simulink model "EXP_Controller_YAW"  (R2015b)
settings: Solver=FixedStepAuto  StartTime=0.0  StopTime=inf  FixedStep=0.1  RelTol=1e-3
values from neighbouring files (symbols this model uses):
  breakpoints1 = data(end:-1:1,1)'    [Experimental_Impl.m]    (also in Experimental_Impl_wPlot.m; FEB02_LAKE_TEST.m; FEB14_LAKE_TEST.m; FEB28_LAKE_TEST.m)
  drag_coeff = 16.91    [Experimental_Impl.m]    (also in Experimental_Impl_wPlot.m; FEB02_LAKE_TEST.m = 8.5; FEB02_Post_Processing.m; FEB14_LAKE_TEST.m)
  Kdy = .1    (= 0.1)    [Experimental_Impl.m]    (also in Experimental_Impl_wPlot.m = Gain(3,i); FEB02_LAKE_TEST.m = 20; FEB02_Post_Processing.m = Gain_Y(3,k); FEB14_LAKE_TEST.m = 20)
  Kiy = .01    (= 0.01)    [Experimental_Impl.m]    (also in Experimental_Impl_wPlot.m = Gain(2,i); FEB02_LAKE_TEST.m; FEB02_Post_Processing.m = Gain_Y(2,k); FEB14_LAKE_TEST.m)
  Kpy = 1    [Experimental_Impl.m]    (also in Experimental_Impl_wPlot.m = Gain(1,i); FEB02_LAKE_TEST.m = 100; FEB02_Post_Processing.m = Gain_Y(1,k); FEB14_LAKE_TEST.m = 100)
  switch_case = 0    [Experimental_Impl.m]    (also in Experimental_Impl_wPlot.m; FEB02_LAKE_TEST.m = 1; FEB02_Post_Processing.m; FEB14_LAKE_TEST.m)
  table_data = data(end:-1:1,2)'    [Experimental_Impl.m]    (also in Experimental_Impl_wPlot.m; FEB02_LAKE_TEST.m; FEB14_LAKE_TEST.m; FEB28_LAKE_TEST.m)
  vf = 0.0    (= 0)    [Experimental_Impl.m]    (also in Experimental_Impl_wPlot.m; FEB02_LAKE_TEST.m = 1.5; FEB02_Post_Processing.m = 1.25; FEB14_LAKE_TEST.m = 1.5)
  vo = 0.0    (= 0)    [Experimental_Impl.m]    (also in Experimental_Impl_wPlot.m; FEB02_LAKE_TEST.m = 1.25; FEB02_Post_Processing.m = 1.25; FEB14_LAKE_TEST.m = 1.25)
  yf = pi/4    (= 0.785398163397)    [Experimental_Impl.m]    (also in Experimental_Impl_wPlot.m = 0; FEB02_LAKE_TEST.m = 0; FEB02_Post_Processing.m = pi()/4; FEB14_LAKE_TEST.m = 0)
  yo = 0    [Experimental_Impl.m]    (also in Experimental_Impl_wPlot.m; FEB02_LAKE_TEST.m; FEB02_Post_Processing.m; FEB14_LAKE_TEST.m)
undefined symbols (not defined in the file or in its folder): Left, Right
libraries: robotlib x3, simulink_extras x3, realtime_pacer_lib x1
settings Model: Creator=bsb  LastModifiedBy=aschnieders22
settings ConfigComp: CovModelRefEnable=Off

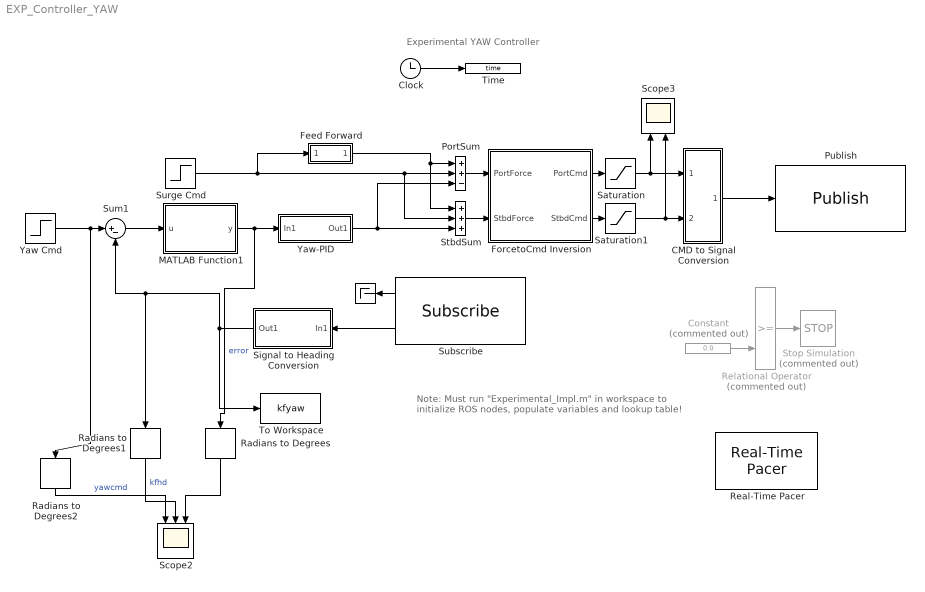
== system EXP_Controller_YAW ==
  note: Note: Must run "Experimental_Impl.m" in workspace to initialize ROS nodes, populate variables and lookup table!
  note: Experimental YAW Controller
  " " : Terminator
  CMD to Signal Conversion : Subsystem
  Clock : Clock
  Constant : Constant  Commented=on  Value=0.0
  Feed Forward : Subsystem
  ForcetoCmd Inversion : Subsystem
  MATLAB Function1 : MATLAB Function  TreatAsAtomicUnit=on
  PortSum : Sum  Inputs=++-
  Publish : robotlib/Publish  SourceLibraryInfo=This block requires Robotics System Toolbox  topicSource=Select from ROS network  topic=/cmd_drive  messageType=kingfisher_msgs/Drive  messageQueueLength=1
  Radians to Degrees : simulink_extras/Transformations/Radians to Degrees
  Radians to Degrees1 : simulink_extras/Transformations/Radians to Degrees
  Radians to Degrees2 : simulink_extras/Transformations/Radians to Degrees
  Real-Time Pacer : realtime_pacer_lib/Real-Time Pacer  simTimePerRealTime=1
  Relational Operator : RelationalOperator  Commented=on  OutDataTypeStr=boolean
  Saturation : Saturate  UpperLimit=1  LowerLimit=-1
  Saturation1 : Saturate  UpperLimit=1  LowerLimit=-1
  Scope2 : Scope  NumInputPorts=3
  Scope3 : Scope  NumInputPorts=2
  Signal to Heading Conversion : Subsystem
  StbdSum : Sum  Inputs=+++
  Stop Simulation : Stop  Commented=on
  Subscribe : robotlib/Subscribe  SourceLibraryInfo=This block requires Robotics System Toolbox  topicSource=Select from ROS network  topic=/imu/data  messageType=sensor_msgs/Imu  sampleTime=-1  messageQueueLength=1
  Sum1 : Sum  Inputs=|+-
  Surge Cmd : Step  Before=vo  After=vf  SampleTime=0
  Time : ToWorkspace  VariableName=time  SampleTime=-1
  To Workspace : ToWorkspace  VariableName=kfyaw  SampleTime=-1
  Yaw Cmd : Step  Time=0  Before=yo  After=yf  SampleTime=0
  Yaw-PID : Subsystem
  wires:
  Clock/1 -> Time/1
  CMD to Signal Conversion/1(Out1) -> Publish/1
  Feed Forward/1(Out1) -> PortSum/1, StbdSum/1
  Saturation1/1 -> Scope3/2, CMD to Signal Conversion/2(In2)
  Saturation/1 -> Scope3/1, CMD to Signal Conversion/1(In1)
  ForcetoCmd Inversion/2(StbdCmd) -> Saturation1/1
  ForcetoCmd Inversion/1(PortCmd) -> Saturation/1
  Subscribe/2 -> Signal to Heading Conversion/1(In1)
  Subscribe/1 -> " "/1
  Yaw-PID/1(Out1) -> StbdSum/3, PortSum/3
  Yaw Cmd/1 -> Radians to Degrees2/1, Sum1/1
  Surge Cmd/1 -> Feed Forward/1(In1), StbdSum/2, PortSum/2
  Sum1/1 -> MATLAB Function1/1(u)
  StbdSum/1 -> ForcetoCmd Inversion/2(StbdForce)
  PortSum/1 -> ForcetoCmd Inversion/1(PortForce)
  Relational Operator/1 -> Stop Simulation/1
  Constant/1 -> Relational Operator/2
  MATLAB Function1/1(y) -> Radians to Degrees/1, Yaw-PID/1(In1)  "error"
  Signal to Heading Conversion/1(Out1) -> Radians to Degrees1/1, Sum1/2, To Workspace/1
  Radians to Degrees1/1 -> Scope2/2  "kfhd"
  Radians to Degrees2/1 -> Scope2/1  "yawcmd"
  Radians to Degrees/1 -> Scope2/3

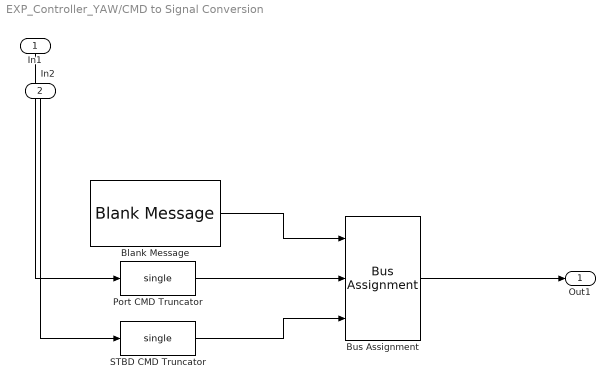
== system EXP_Controller_YAW/CMD to Signal Conversion ==
  In1 : Inport
  In2 : Inport  Port=2
  Blank Message : robotlib/Blank Message  SourceLibraryInfo=This block requires Robotics System Toolbox  messageType=kingfisher_msgs/Drive  SampleTime=inf
  Bus Assignment : BusAssignment  AssignedSignals=Left,Right
  Port CMD Truncator : DataTypeConversion  OutDataTypeStr=single
  STBD CMD Truncator : DataTypeConversion  OutDataTypeStr=single
  Out1 : Outport
  wires:
  In2/1 -> STBD CMD Truncator/1
  In1/1 -> Port CMD Truncator/1
  Bus Assignment/1 -> Out1/1
  Blank Message/1 -> Bus Assignment/1
  Port CMD Truncator/1 -> Bus Assignment/2
  STBD CMD Truncator/1 -> Bus Assignment/3

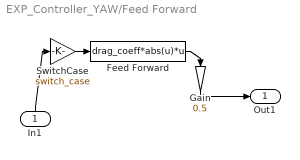
== system EXP_Controller_YAW/Feed Forward ==
  In1 : Inport
  Feed Forward : Fcn  Expr=drag_coeff*abs(u)*u
  Gain : Gain  Gain=0.5
  SwitchCase : Gain  Gain=switch_case
  Out1 : Outport
  wires:
  In1/1 -> SwitchCase/1
  SwitchCase/1 -> Feed Forward/1
  Feed Forward/1 -> Gain/1
  Gain/1 -> Out1/1

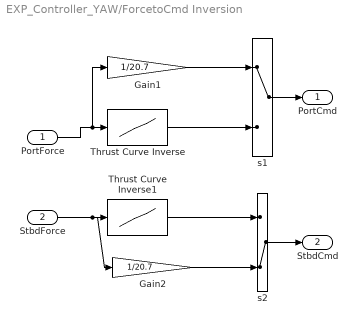
== system EXP_Controller_YAW/ForcetoCmd Inversion ==
  PortForce : Inport
  StbdForce : Inport  Port=2
  Gain1 : Gain  Gain=1/20.7
  Gain2 : Gain  Gain=1/20.7
  Thrust Curve Inverse : Lookup_n-D  NumberOfTableDimensions=1  BreakpointsForDimension1=table_data  Table=breakpoints1  ExtrapMethod=Clip  UseLastTableValue=on  InternalRulePriority=Speed  RndMeth=Simplest  InputSameDT=on
  Thrust Curve Inverse1 : Lookup_n-D  NumberOfTableDimensions=1  BreakpointsForDimension1=table_data  Table=breakpoints1  ExtrapMethod=Clip  UseLastTableValue=on  InternalRulePriority=Speed  RndMeth=Simplest  InputSameDT=on
  "s1 " : ManualSwitch
  s2 : ManualSwitch  CurrentSetting=0
  PortCmd : Outport
  StbdCmd : Outport  Port=2
  wires:
  StbdForce/1 -> Gain2/1, Thrust Curve Inverse1/1
  PortForce/1 -> Gain1/1, Thrust Curve Inverse/1
  Thrust Curve Inverse/1 -> "s1 "/2
  Gain1/1 -> "s1 "/1
  "s1 "/1 -> PortCmd/1
  s2/1 -> StbdCmd/1
  Thrust Curve Inverse1/1 -> s2/1
  Gain2/1 -> s2/2

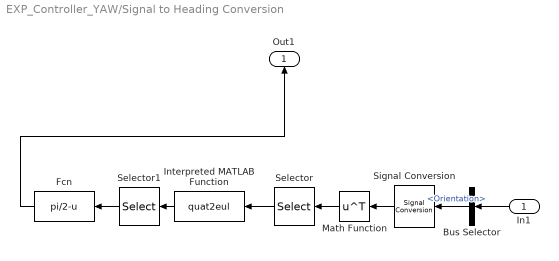
== system EXP_Controller_YAW/Signal to Heading Conversion ==
  In1 : Inport
  Bus Selector : BusSelector  OutputSignals=Orientation
  Fcn : Fcn  Expr=pi/2-u
  Interpreted MATLAB Function : MATLABFcn  MATLABFcn=quat2eul  OutputDimensions=3
  Math Function : Math  Operator=transpose  SaturateOnIntegerOverflow=on
  Selector : Selector  InputPortWidth=4  IndexOptions=Index vector (dialog)  Indices=[4 1 2 3]  OutputSizes=1
  Selector1 : Selector  InputPortWidth=3  IndexOptions=Index vector (dialog)  Indices=1  OutputSizes=1
  Signal Conversion : SignalConversion  ConversionOutput=Virtual bus
  Out1 : Outport
  wires:
  In1/1 -> Bus Selector/1
  Bus Selector/1 -> Signal Conversion/1  "<Orientation>"
  Signal Conversion/1 -> Math Function/1
  Math Function/1 -> Selector/1
  Selector/1 -> Interpreted MATLAB Function/1
  Interpreted MATLAB Function/1 -> Selector1/1
  Selector1/1 -> Fcn/1
  Fcn/1 -> Out1/1

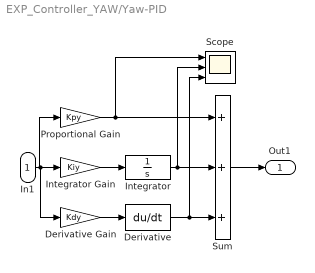
== system EXP_Controller_YAW/Yaw-PID ==
  In1 : Inport
  Derivative : Derivative  CoefficientInTFapproximation=0
  Derivative Gain : Gain  Gain=Kdy
  Integrator : TransferFcn  Denominator=[1 0]
  Integrator Gain : Gain  Gain=Kiy
  Proportional Gain : Gain  Gain=Kpy
  Scope : Scope  NumInputPorts=3
  Sum : Sum  Inputs=+++
  Out1 : Outport
  wires:
  Derivative Gain/1 -> Derivative/1
  Integrator Gain/1 -> Integrator/1
  Derivative/1 -> Scope/3, Sum/3
  Sum/1 -> Out1/1
  Integrator/1 -> Scope/2, Sum/2
  Proportional Gain/1 -> Scope/1, Sum/1
  In1/1 -> Derivative Gain/1, Integrator Gain/1, Proportional Gain/1

== matlab function EXP_Controller_YAW/MATLAB Function1 ==
  data: u input; y output
function y = wrapToPi(u)
%#codegen
while u>pi
    u = u -2*pi;
end;
while u < -pi
    u = u + 2*pi;
end;
y = u;
